simulink model "dcdc1"  (Simulink 8.5)
settings: Solver=ode23tb  StartTime=0.0  StopTime=0.1  FixedStep=1e-8  RelTol=1e-3
libraries: powerlib x17
settings Model: Creator=kmathew  LastModifiedBy=Ratish Kumar S
settings DebuggingCC: SolverPrmCheckMsg=warning  FcnCallInpInsideContextMsg=UseLocalSettings

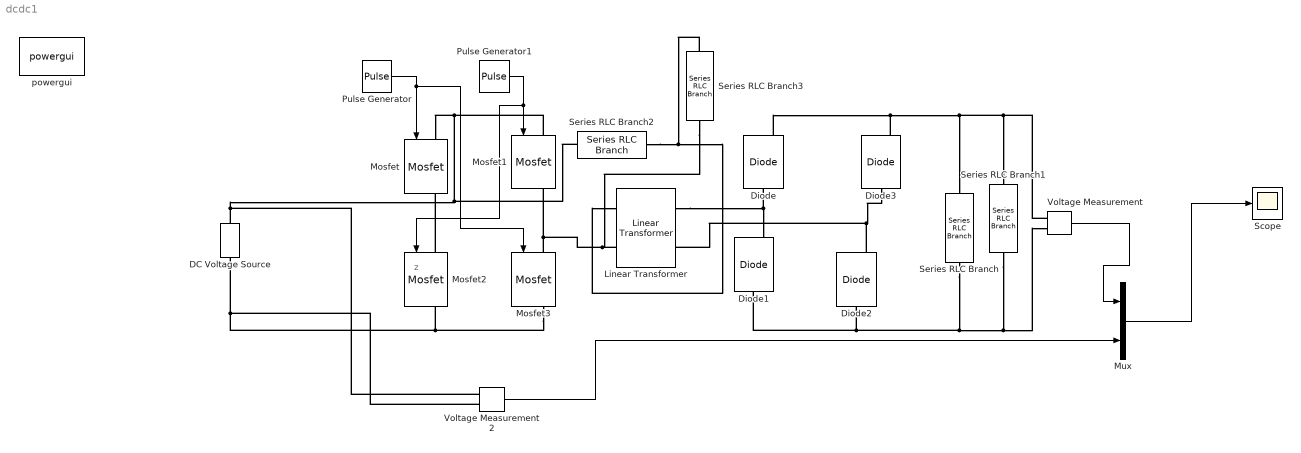
== system dcdc1 ==
  note: z
  DC Voltage Source : powerlib/Electrical Sources/DC Voltage Source  Amplitude=230  Measurements=None
  Diode{,1..3} (4 alike) : powerlib/Power Electronics/Diode  Ron=0.001  Lon=0  Vf=0.8  IC=0  UseSnubber=off  Rs=500  Cs=250e-9  Measurements=on
  Linear Transformer : powerlib/Elements/Linear Transformer  UNITS=SI  NominalPower=[8e3 20000 ]  winding1=[100 0.00025 0]  winding2=[486 0.0004 0]  ThreeWindings=off  winding3=[3.15e+05 24806 7.8961]  RmLm=[1000 21.518e-6]  Measurements=None  DataType=on
  Mosfet{,1..3} (4 alike) : powerlib/Power Electronics/Mosfet  Ron=2e-3  Lon=0  Rd=2e-3  Vfd=1  IC=0  Rs=1e5  Cs=inf  Measurements=on
  Mux : Mux  Inputs=2
  Pulse Generator : DiscretePulseGenerator  PulseType=Time based  Amplitude=5  Period=50e-6  PulseWidth=50
  Pulse Generator1 : DiscretePulseGenerator  PulseType=Time based  Amplitude=5  Period=50e-6  PulseWidth=50  PhaseDelay=25e-6
  Scope : Scope
      settings: YMin=165  YMax=230  Decimation=20
  Series RLC Branch : powerlib/Elements/Series RLC Branch  LConnTagsString=__new0  RConnTagsString=__new0  BranchType=C  Resistance=1  Inductance=1e-3  SetiL0=off  InitialCurrent=0  Capacitance=6.2e-6  Setx0=off  InitialVoltage=0  Measurements=Branch voltage
  Series RLC Branch1 : powerlib/Elements/Series RLC Branch  LConnTagsString=__new0  RConnTagsString=__new0  BranchType=R  Resistance=85.47  Inductance=1e-3  SetiL0=off  InitialCurrent=0  Capacitance=10e-6  Setx0=off  InitialVoltage=0  Measurements=Branch voltage
  Series RLC Branch2 : powerlib/Elements/Series RLC Branch  LConnTagsString=__new0  RConnTagsString=__new0  BranchType=LC  Resistance=100  Inductance=4.06e-6  SetiL0=off  InitialCurrent=0  Capacitance=0.52e-6  Setx0=off  InitialVoltage=0  Measurements=Branch voltage
  Series RLC Branch3 : powerlib/Elements/Series RLC Branch  LConnTagsString=__new0  RConnTagsString=__new0  BranchType=L  Resistance=100  Inductance=21.518e-6  SetiL0=off  InitialCurrent=0  Capacitance=10e-6  Setx0=off  InitialVoltage=0  Measurements=Branch voltage
  Voltage Measurement : powerlib/Measurements/Voltage Measurement  PhasorSimulation=off  OutputType=Complex  PSBequivalent=0
  Voltage Measurement2 : powerlib/Measurements/Voltage Measurement  PhasorSimulation=off  OutputType=Complex  PSBequivalent=0
  powergui : powerlib/powergui  Priority=1  SimulationMode=Continuous  SolverType=Tustin/Backward Euler (TBE)  SampleTime=1e-8  frequency=60  SPID=off  DisableSnubberDevices=off  DisableRonSwitches=off  DisableVfSwitches=off  SwTol=0  DisplayEquations=off  Interpol=off  methode=off  Ts=100  FunctionMessages=off  echomessages=off  HookPort=off  EnableUseOfTLC=off  x0status=blocks  frequencyindice=0  Pbase=100e6  ErrMax=1e-4  Iterations=50  UnitsV=kV  UnitsW=MW  buscounter=0  RestoreLinks=warning  ResistiveCurrentMeasurement=off  Frange=[0:2:500]  Ylog=off  Xlog=on  ShowGrid=off  save=off  variable=ZData  structure=0  ZoomFFT=off  StartTime=0.0  cycles=1  DisplayStyle=1  fundamental=60  FreqAxis=off  MaxFrequency=1000  frequencyindicesteady=1  RmsSteady=1  display=off
  wires:
  Voltage Measurement/1 -> Mux/1
  Pulse Generator/1 -> Mosfet/1, Mosfet3/1
  Pulse Generator1/1 -> Mosfet2/1, Mosfet1/1
  ? -> ?
  Voltage Measurement2/1 -> Mux/2
  Mux/1 -> Scope/1
  connections:
  Linear Transformer/LConn2 -- Mosfet1/RConn1 -- Mosfet3/LConn1 -- Series RLC Branch3/RConn1
  Mosfet1/LConn1 -- Series RLC Branch2/RConn1 -- Voltage Measurement2/LConn1 -- DC Voltage Source/RConn1 -- Mosfet/LConn1
  Mosfet3/RConn1 -- Mosfet2/RConn1 -- DC Voltage Source/LConn1 -- Voltage Measurement2/LConn2
  Diode2/RConn1 -- Linear Transformer/RConn2 -- Diode3/LConn1
  Linear Transformer/RConn1 -- Diode1/RConn1 -- Diode/LConn1
  Series RLC Branch/RConn1 -- Voltage Measurement/LConn2 -- Series RLC Branch1/RConn1 -- Diode2/LConn1 -- Diode1/LConn1
  Voltage Measurement/LConn1 -- Diode3/RConn1 -- Diode/RConn1 -- Series RLC Branch/LConn1 -- Series RLC Branch1/LConn1
  Mosfet2/LConn1 -- Mosfet/RConn1
  Series RLC Branch2/LConn1 -- Linear Transformer/LConn1 -- Series RLC Branch3/LConn1
